simulink model "positionControl"  (Simulink 8.7)
settings: Solver=FixedStepDiscrete  StartTime=0.0  StopTime=SIMULATION_TIME  FixedStep=ts  RelTol=1e-3
values from neighbouring files (symbols this model uses):
  qjDes = zeros(length(res)-1-cuttingStep,15)    [getDataFromTxt.m]
  time = zeros(length(res)-1-cuttingStep,1)    [getDataFromTxt.m]
libraries: WBToolboxLibrary x4
settings Model: Creator=DanielePucci  LastModifiedBy=gnava
settings DataIOCC: LimitDataPoints=off  SaveFormat=Dataset
settings DebuggingCC: UnderspecifiedInitializationDetection=Simplified  MergeDetectMultiDrivingBlocksExec=error
settings HardwareCC: ProdBitPerPointer=64  ProdLargestAtomicFloat=Float  ProdIntDivRoundTo=Zero  ProdEndianess=LittleEndian  ProdWordSize=64  ProdHWDeviceType=Intel->x86-64 (Windows64)
settings ModelReferenceCC: PropagateSignalLabelsOutOfModel=on
settings ConfigComp: CovModelRefEnable=off

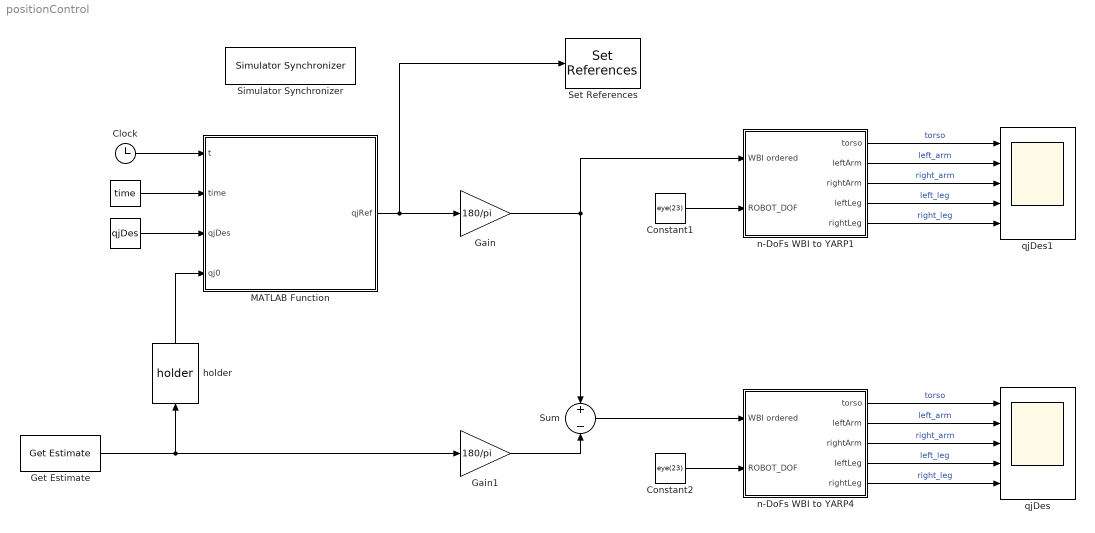
== system positionControl ==
  "   " : Constant  Value=qjDes
  "               " : Constant  Value=time
  Clock : Clock
  Constant1 : Constant  Value=eye(23)
  Constant2 : Constant  Value=eye(23)
  Gain : Gain  Gain=180/pi
  Gain1 : Gain  Gain=180/pi
  Get Estimate : WBToolboxLibrary/wholeBodyStates/Get Estimate  estimateType=Joints Position  robotName=WBT_robotName  localName=WBT_modelName  wbiFile=WBT_wbiFilename  wbiList=WBT_wbiList
  MATLAB Function : MATLAB Function  TreatAsAtomicUnit=on
  Set References : WBToolboxLibrary/wholeBodyActuators/Set References  controlType=Position Direct  robotName=WBT_robotName  localName=WBT_modelName  wbiFile=WBT_wbiFilename  wbiList=WBT_wbiList
  Simulator Synchronizer : WBToolboxLibrary/Utilities/Simulator Synchronizer  period=ts  serverPortName='/clock/rpc'  clientPortName='/WBT_synchronizer/rpc:o'
  Sum : Sum  Inputs=+-
  "holder " : WBToolboxLibrary/Utilities/holder 
  n-DoFs WBI to YARP1 : Subsystem
  n-DoFs WBI to YARP4 : Subsystem
  qjDes : Scope  NumInputPorts=5
  qjDes1 : Scope  NumInputPorts=5
  wires:
  "               "/1 -> MATLAB Function/2(time)
  Clock/1 -> MATLAB Function/1(t)
  "   "/1 -> MATLAB Function/3(qjDes)
  Sum/1 -> n-DoFs WBI to YARP4/1(WBI ordered)
  n-DoFs WBI to YARP4/4(leftLeg) -> qjDes/4  "left_leg"
  n-DoFs WBI to YARP4/5(rightLeg) -> qjDes/5  "right_leg"
  n-DoFs WBI to YARP4/3(rightArm) -> qjDes/3  "right_arm"
  n-DoFs WBI to YARP4/1(torso) -> qjDes/1  "torso"
  n-DoFs WBI to YARP4/2(leftArm) -> qjDes/2  "left_arm"
  Get Estimate/1 -> "holder "/1, Gain1/1
  Constant2/1 -> n-DoFs WBI to YARP4/2(ROBOT_DOF)
  n-DoFs WBI to YARP1/4(leftLeg) -> qjDes1/4  "left_leg"
  n-DoFs WBI to YARP1/5(rightLeg) -> qjDes1/5  "right_leg"
  n-DoFs WBI to YARP1/3(rightArm) -> qjDes1/3  "right_arm"
  n-DoFs WBI to YARP1/1(torso) -> qjDes1/1  "torso"
  n-DoFs WBI to YARP1/2(leftArm) -> qjDes1/2  "left_arm"
  Constant1/1 -> n-DoFs WBI to YARP1/2(ROBOT_DOF)
  MATLAB Function/1(qjRef) -> Set References/1, Gain/1
  Gain1/1 -> Sum/2
  Gain/1 -> n-DoFs WBI to YARP1/1(WBI ordered), Sum/1
  "holder "/1 -> MATLAB Function/4(qj0)

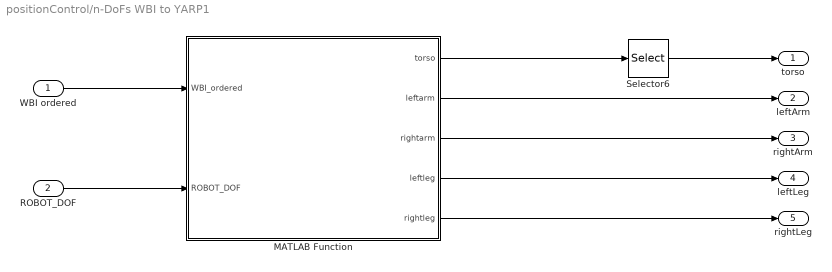
== system positionControl/n-DoFs WBI to YARP1 ==
  WBI ordered : Inport
  ROBOT_DOF : Inport  Port=2
  MATLAB Function : MATLAB Function  TreatAsAtomicUnit=on
  Selector6 : Selector  InputPortWidth=3  IndexOptions=Index vector (dialog)  Indices=[3 2 1]  OutputSizes=1
  torso : Outport
  leftArm : Outport  Port=2
  rightArm : Outport  Port=3
  leftLeg : Outport  Port=4
  rightLeg : Outport  Port=5
  wires:
  Selector6/1 -> torso/1
  MATLAB Function/1(torso) -> Selector6/1
  WBI ordered/1 -> MATLAB Function/1(WBI_ordered)
  ROBOT_DOF/1 -> MATLAB Function/2(ROBOT_DOF)
  MATLAB Function/2(leftarm) -> leftArm/1
  MATLAB Function/3(rightarm) -> rightArm/1
  MATLAB Function/4(leftleg) -> leftLeg/1
  MATLAB Function/5(rightleg) -> rightLeg/1

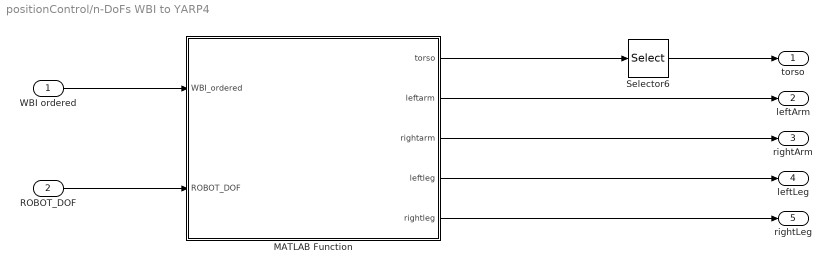
== system positionControl/n-DoFs WBI to YARP4 ==
  WBI ordered : Inport
  ROBOT_DOF : Inport  Port=2
  MATLAB Function : MATLAB Function  TreatAsAtomicUnit=on
  Selector6 : Selector  InputPortWidth=3  IndexOptions=Index vector (dialog)  Indices=[3 2 1]  OutputSizes=1
  torso : Outport
  leftArm : Outport  Port=2
  rightArm : Outport  Port=3
  leftLeg : Outport  Port=4
  rightLeg : Outport  Port=5
  wires:
  Selector6/1 -> torso/1
  MATLAB Function/1(torso) -> Selector6/1
  WBI ordered/1 -> MATLAB Function/1(WBI_ordered)
  ROBOT_DOF/1 -> MATLAB Function/2(ROBOT_DOF)
  MATLAB Function/2(leftarm) -> leftArm/1
  MATLAB Function/3(rightarm) -> rightArm/1
  MATLAB Function/4(leftleg) -> leftLeg/1
  MATLAB Function/5(rightleg) -> rightLeg/1

== matlab function n-DoFs WBI to YARP1/MATLAB Function ==
  data: WBI_ordered input double; torso output double; ROBOT_DOF input double; leftarm output double; rightarm output double; leftleg output double; rightleg output double
function [torso,leftarm,rightarm,leftleg,rightleg] = increaseDofTo25ForVisualizer(WBI_ordered,ROBOT_DOF)

% codeGen
[torso,leftarm,rightarm,leftleg,rightleg] = increaseDofTo25ForVisualizer(WBI_ordered,ROBOT_DOF);

end

== matlab function MATLAB Function ==
  data: t input double; time input double; qjRef output double; qjDes input double; qj0 input double
function qjRef  = generateReferences(t,time,qjDes,qj0) 

i     = 0;
qjRef = qj0;
eps   = 0.001;

for k = 1:length(time)
    
    if  t>time(k)-eps && t<time(k)+eps
        
       i = k;
    end
end

qjRef([18 19 21 22]) = qjDes(i,1:4);
qjRef([12 13 15 16]) = qjDes(i,1:4);
qjRef([8 9 10 11])   = qjDes(i,5:8);
qjRef([4 5 6 7])     = qjDes(i,5:8);
qjRef(1)             = qjDes(i,9);

end

== matlab function n-DoFs WBI to YARP4/MATLAB Function ==
  data: WBI_ordered input double; torso output double; ROBOT_DOF input double; leftarm output double; rightarm output double; leftleg output double; rightleg output double
function [torso,leftarm,rightarm,leftleg,rightleg] = increaseDofTo25ForVisualizer(WBI_ordered,ROBOT_DOF)

% codeGen
[torso,leftarm,rightarm,leftleg,rightleg] = increaseDofTo25ForVisualizer(WBI_ordered,ROBOT_DOF);

end
